simulink model "n98tot98reg60neu"  (R2023b)
settings: Solver=VariableStepAuto  StartTime=0.0  StopTime=10.0  RelTol=1e-3
libraries: neural x66
(part 3 of 3)

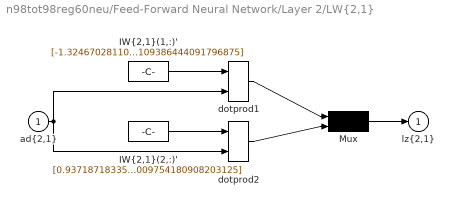
== system n98tot98reg60neu/Feed-Forward Neural Network/Layer 2/LW{2,1} ==
  "ad{2,1}" : Inport  PortDimensions=60
      mask Display: e = 0.06;c1 = [120 230 180]/255;c2 = ([120 230 180]+0)/(256+128);c3 = ([120 230 180]+128)/(256+128);patch([0 1 1 0],[0 0 1 1],c1);patch([0 1 1 1-e 1-e 0+e],[0 0 1 1-e 0+e 0+e],c2);patch([0 0 1 1-e 0+e 0+e],[0 1 1 1-e 1-e 0+e],c3);plot([0 1 1 0 0],[0 0 1 1 0]);
  "IW{2,1}(1,:)'" : Constant  Value=[-1.3246702811010473421760025303228758275508880615234375;-0.0943084688819128269532399144736700691282749176025390625;-0.042144241538095976451483437585920910350978374481201171875;-1.3799411102722631827788291047909297049045562744140625;-0.82454702197546314579312820569612085819244384765625;-0.0925502818312342878659393363705021329224109649658203125;-0.84031205644009732136368029387085698544979095458984375;1.01084907372054733087907152366824448108673095703125;-0.456342166698917750533581738636712543666362762451171875;-0.57313010933097230381605413640500046312808990478515625;-0.46257745235969049968360877755912952125072479248046875;0.213006506437510012563762984427739866077899932861328125;0.301675891573022048053331900518969632685184478759765625;1.79452909115708880705142291844822466373443603515625;-1.0027767467578760918200941887334920465946197509765625;-0.52353870157094462012281610441277734935283660888671875;-1.0800871184000282454462649184279143810272216796875;-0.82887931136394754627616521247546188533306121826171875;0.052985323912125459333566368513857014477252960205078125;1.008520958479638185423254981287755072116851806640625;-0.6826481094876168942420235907775349915027618408203125;0.160377501343295814084655148690217174589633941650390625;-0.2401764425828963600562104829805321060121059417724609375;0.9021449160371821651693835519836284220218658447265625;0.6785308712676390019424843558226712048053741455078125;-1.1906886837263124245822609736933372914791107177734375;-0.8137123462582775967888437662622891366481781005859375;1.37334057114164043156279149116016924381256103515625;0.66590450504941467446684555397951044142246246337890625;-0.5493250995555960525251748549635522067546844482421875;-0.77094504802390007025536533546983264386653900146484375;1.0188986033795266461510209410334937274456024169921875;0.860547172518857816925219594850204885005950927734375;1.470357304660392383510725267115049064159393310546875;-0.70764411393360970858878999933949671685695648193359375;0.97114972475294714104876447891001589596271514892578125;-1.6313746343639223823629436083137989044189453125;-0.8720563448523659388911255518905818462371826171875;-0.08728037818226118405018354451385675929486751556396484375;0.360639021498661949127750858679064549505710601806640625;-0.0239218245839044711675835941377954441122710704803466796875;0.387694755795795653607882513824733905494213104248046875;0.61792007422549743989037551727960817515850067138671875;-0.07597915208083694249552308974671177566051483154296875;0.048493613475773238163935019429118256084620952606201171875;0.448572609736800576030191223253495991230010986328125;1.3599434010962834218361194871249608695507049560546875;1.2339731294233755587441692114225588738918304443359375;0.75356049348767417672689816754427738487720489501953125;0.488223512776593315809492423795745708048343658447265625;0.791002916770465080986696193576790392398834228515625;-2.06722866460731946602891184738837182521820068359375;0.68526404447103461681223279811092652380466461181640625;-1.2550570476147206999684158290619961917400360107421875;-0.5857053538945631299128535829368047416210174560546875;-0.90128263208402448203315771024790592491626739501953125;-0.80000170488106314703458110670908354222774505615234375;-0.44936014307566474190736016680602915585041046142578125;0.33501629260751142336260954834870062768459320068359375;0.0210486964157857829593734066975230234675109386444091796875]
      mask Display: e = 0.06;c1 = [120 150 230]/255;c2 = ([120 150 230]+0)/383;c3 = ([120 150 230]+128)/383;patch([0 1 1 0],[0 0 1 1],c1);patch([0 1 1 1-e 1-e 0+e],[0 0 1 1-e 0+e 0+e],c2);patch([0 0 1 1-e 0+e 0+e],[0 1 1 1-e 1-e 0+e],c3);plot([0 1 1 0 0],[0 0 1 1 0]);disp('weights');
  "IW{2,1}(2,:)'" : Constant  Value=[0.9371871833526645989564940464333631098270416259765625;-0.68239009385453031075741137101431377232074737548828125;0.4542415053241881661705292572150938212871551513671875;0.294800789758634940174175653737620450556278228759765625;-0.8131891782526528000829557640827260911464691162109375;0.57747283472109678381656294732238166034221649169921875;0.04739862223319725453851702923202537931501865386962890625;0.1652095695522351193051946438572485931217670440673828125;0.47825282071270691641728944887290708720684051513671875;-0.11754357436768513023306326203964999876916408538818359375;-0.6553738049692545697411105720675550401210784912109375;0.40381281880629860125964114558883011341094970703125;-0.64697538858500192038292198049020953476428985595703125;1.1393951776370354611600532734883017838001251220703125;-0.14510164024711469377137973424396477639675140380859375;0.042077268477991917883240802211730624549090862274169921875;0.1670900127642803989491682159496122039854526519775390625;0.218354613168486089147535267329658381640911102294921875;-0.35085359840563057343132413734565488994121551513671875;0.53476951081162604761942702680244110524654388427734375;-0.213673844565132442507859877878217957913875579833984375;-0.2119295447259303688536391518937307409942150115966796875;-0.415213714100154118735730435219011269509792327880859375;0.321170931685458571624991463977494277060031890869140625;0.59068108418025655481642388622276484966278076171875;0.1993409290031344649474220886986586265265941619873046875;-0.266186683543138069563127601213636808097362518310546875;-0.0711823548010912243722003722723457030951976776123046875;-0.0761741247687779676756036906226654537022113800048828125;-0.150618354606124660310939589180634357035160064697265625;0.2249919748330519164714047519737505353987216949462890625;0.514507307761812970881010187440551817417144775390625;0.267187855660000861401925931204459629952907562255859375;-0.1163986941711229461393628525911481119692325592041015625;-0.55190670988247603201415358853409998118877410888671875;-0.07859445421403078724242874386618495918810367584228515625;-0.5948567496515682062607766056316904723644256591796875;0.73426059100503682230964841437526047229766845703125;0.521933019146352261685706253047101199626922607421875;-0.387288977289993063823914098975365050137042999267578125;-0.6991444888640925281464433282963000237941741943359375;-0.5232626561327566871995031760889105498790740966796875;0.73028293604696992158409329931600950658321380615234375;0.382157944235874069693892352006514556705951690673828125;-0.96256246443723758599020356996334157884120941162109375;0.31262913541236592163130580956931225955486297607421875;0.539036458335544477193934653769247233867645263671875;-0.15338974821037731910422508008196018636226654052734375;-0.36767494828096591863442199610290117561817169189453125;-0.06345365939536863619796491775559843517839908599853515625;-0.451767561211840362744851518073119223117828369140625;0.3426984067374245768178298021666705608367919921875;-0.503408613431348239686258239089511334896087646484375;0.86283532695471831797107142847380600869655609130859375;0.70606837065722327650973966228775680065155029296875;0.317565875803807851074367363253259100019931793212890625;-0.54520168748265074309955480202916078269481658935546875;-0.59662276924797208454975816493970341980457305908203125;0.7942800818688195985117772579542361199855804443359375;-0.1774995877005108024793145204967004247009754180908203125]
      mask Display: e = 0.06;c1 = [120 150 230]/255;c2 = ([120 150 230]+0)/383;c3 = ([120 150 230]+128)/383;patch([0 1 1 0],[0 0 1 1],c1);patch([0 1 1 1-e 1-e 0+e],[0 0 1 1-e 0+e 0+e],c2);patch([0 0 1 1-e 0+e 0+e],[0 1 1 1-e 1-e 0+e],c3);plot([0 1 1 0 0],[0 0 1 1 0]);disp('weights');
  Mux : Mux  Inputs=2
      mask Display: e = 0.06;c1 = [120 150 230]/255;c2 = ([120 150 230]+0)/383;c3 = ([120 150 230]+128)/383;patch([0 1 1 0],[0 0 1 1],c1);patch([0 1 1 1-e 1-e 0+e],[0 0 1 1-e 0+e 0+e],c2);patch([0 0 1 1-e 0+e 0+e],[0 1 1 1-e 1-e 0+e],c3);plot([0 1 1 0 0],[0 0 1 1 0]);disp('Mux');
  dotprod1 : neural/Weight Functions/dotprod
  dotprod2 : neural/Weight Functions/dotprod
  "lz{2,1}" : Outport
      mask Display: e = 0.06;c1 = [120 230 180]/255;c2 = ([120 230 180]+0)/(256+128);c3 = ([120 230 180]+128)/(256+128);patch([0 1 1 0],[0 0 1 1],c1);patch([0 1 1 1-e 1-e 0+e],[0 0 1 1-e 0+e 0+e],c2);patch([0 0 1 1-e 0+e 0+e],[0 1 1 1-e 1-e 0+e],c3);plot([0 1 1 0 0],[0 0 1 1 0]);
  wires:
  "IW{2,1}(1,:)'"/1 -> dotprod1/1
  "ad{2,1}"/1 -> dotprod1/2, dotprod2/2
  dotprod1/1 -> Mux/1
  "IW{2,1}(2,:)'"/1 -> dotprod2/1
  dotprod2/1 -> Mux/2
  Mux/1 -> "lz{2,1}"/1
